simulink model "Struct"  (R2023b)
settings: Solver=VariableStepAuto  StartTime=0.0  StopTime=5  FixedStep=1e-3  MaxStep=1e-3  RelTol=1e-3
values from neighbouring files (symbols this model uses):
  d_1 = 19.4    [CONSTANTS.m]
  d_2 = 24.7    [CONSTANTS.m]
  Ixx_1 = 9.4    [CONSTANTS.m]
  Ixx_2 = 16.5    [CONSTANTS.m]
  Iyy_1 = 9.4    [CONSTANTS.m]
  Iyy_2 = 16.5    [CONSTANTS.m]
  Izz_1 = 0.7    [CONSTANTS.m]
  Izz_2 = 0.7    [CONSTANTS.m]
  Izz_3 = 9.1    [CONSTANTS.m]
  K1_1 = 38.80    (= 38.8)    [CONSTANTS.m]
  K1_2 = 23.30    (= 23.3)    [CONSTANTS.m]
  K2_1 = 2.94    [CONSTANTS.m]
  K2_2 = 2.8    [CONSTANTS.m]
  K3_1 = 9.6    [CONSTANTS.m]
  K3_2 = 11.7    [CONSTANTS.m]
  K4_1 = 0.044    [CONSTANTS.m]
  K4_2 = 0.043    [CONSTANTS.m]
  K5_1 = 15.6    [CONSTANTS.m]
  K5_2 = 9.4    [CONSTANTS.m]
  l_1 = 0.55    [CONSTANTS.m]
  l_2 = 0.55    [CONSTANTS.m]
  m_1 = 46    [CONSTANTS.m]
  m_2 = 78    [CONSTANTS.m]
  x_block = 0.1    [CONSTANTS.m]
  y_block = 0.1    [CONSTANTS.m]
  z_block = 0.1    [CONSTANTS.m]
undefined symbols (not defined in the file or in its folder): X, Y, Z
libraries: sm_lib x19, nesl_utility x13
settings Model: Creator=ycheb  LastModifiedBy=ycheb
settings ExplorerConfigSet: InternalSimMechanicsExplorerSettings="<ExplorerConfiguration><canonicalview>default</canonicalview><AnimationSetting><BasePlaybackSpeed>1.0</BasePlaybackSpeed><PlaybackSpeedFactor>1.0</PlaybackSpeedFactor></AnimationSetting><TilePanel><TileInfo><Tiles Columns=\"1\" Count=\"1\" Rows=\"1\"><Column Weight=\"1\"/><Row Weight=\"1\"/><Tile Height=\"1\" Width=\"1\" X=\"0\" Y=\"0\"/></Tiles></TileInfo><SceneInfo><SceneViewer><BGColor><R>0.60000002384185791</R><G>0.60000002384185791</G><B>0.60000002384185791</B></BGColor><Camera><DoPerspective>off</DoPerspective><Position><X>0.167180391738689205</X><Y>-1.3498377752304076</Y><Z>-0.780521391542822407</Z></Position><Center><X>0.167180391738689205</X><Y>2.22044604925031308e-16</Y><Z>-0.780521391542822407</Z></Center><Up><X>0</X><Y>-0</Y><Z>1</Z></Up><ViewLimDist>1</ViewLimDist><YLim>1.46214565410614039</YLim><XLim>3.24130518896980702</XLim></Camera></SceneViewer></SceneInfo></TilePanel><MechEditorPanel><Cameras/><GfxPanelCameraMap/><VideoCreator><PlaybackSpeedRatio>1.0</PlaybackSpeedRatio><FrameRate>30</FrameRate><VideoFormat>Motion JPEG AVI</VideoFormat><FrameSize>[1280 720]</FrameSize></VideoCreator></MechEditorPanel></ExplorerConfiguration>"

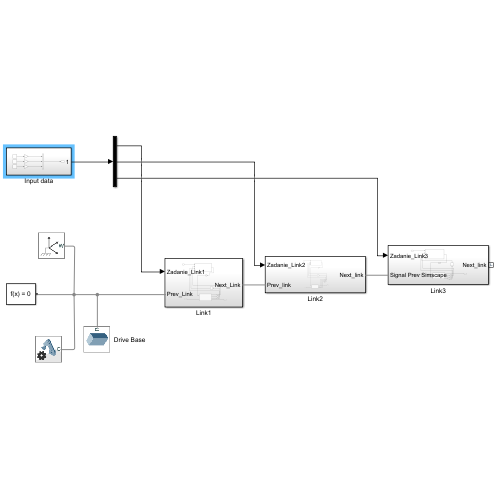
[thumbnail: Simulink's stored preview of the top-level diagram]
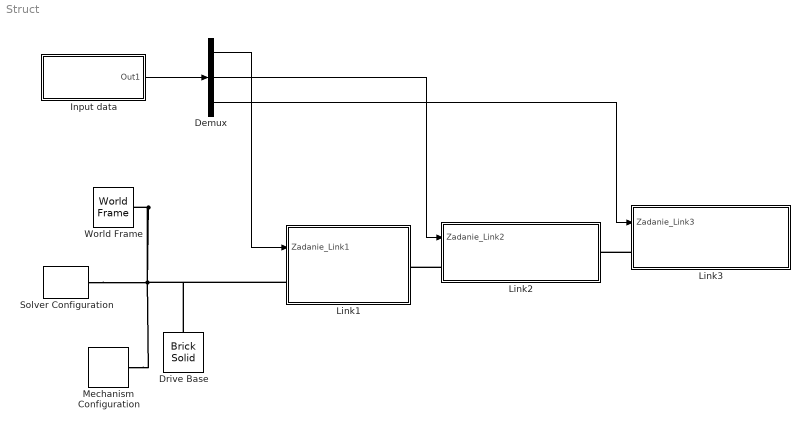
== system Struct ==
  Demux : Demux  Outputs=3
  Drive Base : sm_lib/Body Elements/Brick Solid  GraphicAmbientColor=[0.15 0.15 0.15 1.0]  BasedOnType=Density  BrickDimensions=[x_block y_block z_block]  BrickDimensionsUnits=m  CenterOfMass=[0 0 0]  CenterOfMassUnits=m  GraphicDiffuseColor=[0.5 0.5 0.5]  Density=1000  DensityUnits=kg/m^3  DoExposeReferenceFrame=on  GraphicEmissiveColor=[0.0 0.0 0.0 1.0]  ExportEntireGeometry=off  SerializedFrames=<Frames/>  MarkerShape=Sphere  MarkerSize=10  GraphicType=FromGeometry  InertiaType=CalculateFromGeometry  Mass=1  MassUnits=kg  MomentsOfInertia=[1 1 1]  MomentsOfInertiaUnits=kg*m^2  GraphicOpacity=1.0  ProductsOfInertia=[0 0 0]  ProductsOfInertiaUnits=kg*m^2  GraphicShininess=75  GraphicSpecularColor=[0.5 0.5 0.5 1.0]  GraphicVisPropType=SimpleVisualProperties
  Input data : Subsystem
  Link1 : Subsystem
  Link2 : Subsystem
  Link3 : Subsystem
  Mechanism Configuration : sm_lib/Utilities/Mechanism Configuration  UniformGravity=Constant  GravityVector=[0 0 -9.80665]  GravityVectorUnits=m/s^2  LinearizationDelta=0.001  JointModeTransitionNonlinearIterations=2
  Solver Configuration : nesl_utility/Solver Configuration  PhysicalDomain=network_engine_domain  SubClassName=solver  LeftPortType=input  RightPortType=generic  Tones=[]  Harmonics=[]  SimulateNoise=off  Profile=off  UseLocalSampling=off  EnableSwitchedLinearOptims=on  FrequencyDomain=off  UseCCode=off  RelTol=0.001  AbsTol=0.001  MinStep=1e-09  ToWorkspace=off  RevertToSquareIcSolve=off  NumHomotopyIterations=100  PhasorMode=off  PhasorModeNumHarmonics=1  ConsistencySolver=NEWTON_XTOL_AFTER_FTOL  IndexReductionMethod=DerivativeReplacement  DoDC=off  ResidualTolerance=1e-09  ConsistencyTolSource=GLOBAL  ConsistencyAbsTol=0.001  ConsistencyRelTol=0.001  ConsistencyTolFactor=0.001  UseLocalSolver=off  LocalSolverChoice=NE_BACKWARD_EULER_ADVANCER  ResolveIndetEquations=on  FunctionEvalNumThread=1  LocalSolverSampleTime=0.001  DoFixedCost=off  MaxNonlinIter=3  MaxModeIter=2  ComputeImpulses=off  ImpulseIterations=2  LinearAlgebra=auto  LinearAlgebraNumThread=0  EquationFormulation=NE_TIME_EF  DelaysMemoryBudget=1024  AutomaticFiltering=on  FilteringTimeConstant=0.001  PartitionStorageMethod=AS_NEEDED  PartitionMemoryBudget=1024  PartitionMethod=ROBUST  MultibodyUseLocalSolver=off  MultibodyLocalSolverChoice=ODE1  MultibodyLocalSolverSampleTime=0.001
  World Frame : sm_lib/Frames and Transforms/World Frame
  wires:
  Demux/1 -> Link1/1(Zadanie_Link1)
  Demux/2 -> Link2/1(Zadanie_Link2)
  Demux/3 -> Link3/1(Zadanie_Link3)
  Input data/1(Out1) -> Demux/1
  connections:
  World Frame/RConn1 -- Drive Base/RConn1 -- Link1/LConn1 -- Solver Configuration/RConn1 -- Mechanism Configuration/RConn1
  Link2/LConn1 -- Link1/RConn1
  Link3/LConn1 -- Link2/RConn1

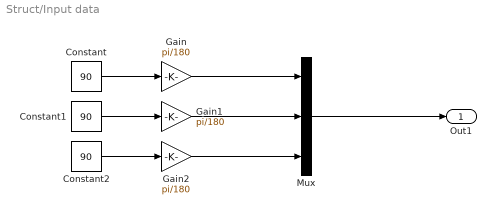
== system Struct/Input data ==
  Constant : Constant  Value=90
  Constant1 : Constant  Value=90
  Constant2 : Constant  Value=90
  Gain : Gain  Gain=pi/180
  Gain1 : Gain  Gain=pi/180
  Gain2 : Gain  Gain=pi/180
  Mux : Mux  Inputs=3
  Out1 : Outport
  wires:
  Mux/1 -> Out1/1
  Constant/1 -> Gain/1
  Constant1/1 -> Gain1/1
  Constant2/1 -> Gain2/1
  Gain/1 -> Mux/1
  Gain1/1 -> Mux/2
  Gain2/1 -> Mux/3

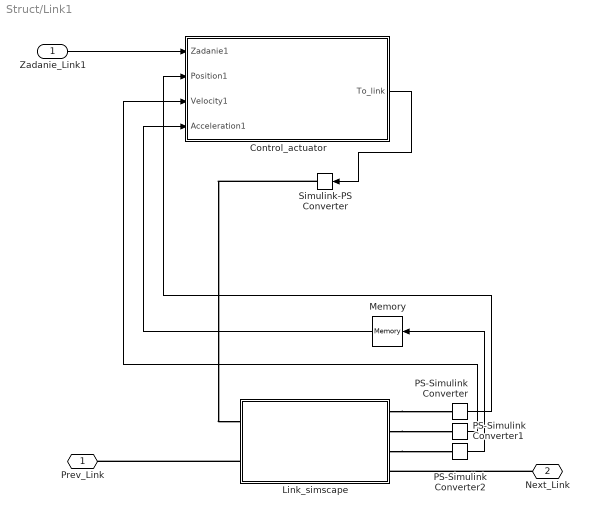
== system Struct/Link1 ==
  Zadanie_Link1 : Inport
  Control_actuator : Subsystem
  Link_simscape : Subsystem
  Memory : Memory
  PS-Simulink Converter : nesl_utility/PS-Simulink Converter  PhysicalDomain=network_engine_domain  SubClassName=ps_output  LeftPortType=input  RightPortType=output  PseudoPeriodic=off  Frequencies=[]  VectorFormat=inherit  Unit=inherit  AffineConversion=off
  PS-Simulink Converter1 : nesl_utility/PS-Simulink Converter  PhysicalDomain=network_engine_domain  SubClassName=ps_output  LeftPortType=input  RightPortType=output  PseudoPeriodic=off  Frequencies=[]  VectorFormat=inherit  Unit=inherit  AffineConversion=off
  PS-Simulink Converter2 : nesl_utility/PS-Simulink Converter  PhysicalDomain=network_engine_domain  SubClassName=ps_output  LeftPortType=input  RightPortType=output  PseudoPeriodic=off  Frequencies=[]  VectorFormat=inherit  Unit=inherit  AffineConversion=off
  Simulink-PS Converter : nesl_utility/Simulink-PS Converter  PhysicalDomain=network_engine_domain  SubClassName=ps_input  LeftPortType=input  RightPortType=output  PseudoPeriodic=off  Frequencies=[]  NoiseDistribution=none  NoiseParameters=[]  Unit=1  AffineConversion=off  FilteringAndDerivatives=provide  SimscapeFilterOrder=1  InputFilterTimeConstant=0.001  UdotUserProvided=0
  Prev_Link : PMIOPort  Side=Left
  Next_Link : PMIOPort  Port=2  Side=Right
  wires:
  Control_actuator/1(To_link) -> Simulink-PS Converter/1
  PS-Simulink Converter/1 -> Control_actuator/2(Position1)
  PS-Simulink Converter1/1 -> Control_actuator/3(Velocity1)
  PS-Simulink Converter2/1 -> Memory/1
  Zadanie_Link1/1 -> Control_actuator/1(Zadanie1)
  Memory/1 -> Control_actuator/4(Acceleration1)
  connections:
  Link_simscape/LConn2 -- Prev_Link/RConn1
  Next_Link/RConn1 -- Link_simscape/RConn4
  Link_simscape/RConn1 -- PS-Simulink Converter/LConn1
  Link_simscape/RConn3 -- PS-Simulink Converter2/LConn1
  Link_simscape/RConn2 -- PS-Simulink Converter1/LConn1
  Simulink-PS Converter/RConn1 -- Link_simscape/LConn1

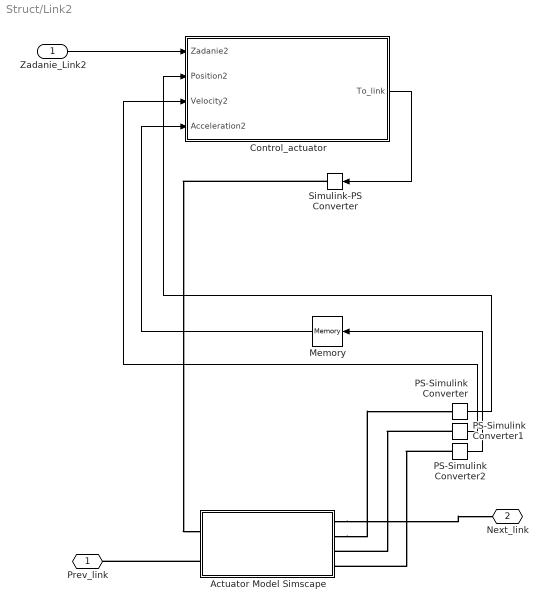
== system Struct/Link2 ==
  Zadanie_Link2 : Inport
  Actuator Model Simscape : Subsystem
  Control_actuator : Subsystem
  Memory : Memory
  PS-Simulink Converter : nesl_utility/PS-Simulink Converter  PhysicalDomain=network_engine_domain  SubClassName=ps_output  LeftPortType=input  RightPortType=output  PseudoPeriodic=off  Frequencies=[]  VectorFormat=inherit  Unit=inherit  AffineConversion=off
  PS-Simulink Converter1 : nesl_utility/PS-Simulink Converter  PhysicalDomain=network_engine_domain  SubClassName=ps_output  LeftPortType=input  RightPortType=output  PseudoPeriodic=off  Frequencies=[]  VectorFormat=inherit  Unit=inherit  AffineConversion=off
  PS-Simulink Converter2 : nesl_utility/PS-Simulink Converter  PhysicalDomain=network_engine_domain  SubClassName=ps_output  LeftPortType=input  RightPortType=output  PseudoPeriodic=off  Frequencies=[]  VectorFormat=inherit  Unit=inherit  AffineConversion=off
  Simulink-PS Converter : nesl_utility/Simulink-PS Converter  PhysicalDomain=network_engine_domain  SubClassName=ps_input  LeftPortType=input  RightPortType=output  PseudoPeriodic=off  Frequencies=[]  NoiseDistribution=none  NoiseParameters=[]  Unit=1  AffineConversion=off  FilteringAndDerivatives=provide  SimscapeFilterOrder=1  InputFilterTimeConstant=0.001  UdotUserProvided=0
  Prev_link : PMIOPort  Side=Left
  Next_link : PMIOPort  Port=2  Side=Right
  wires:
  PS-Simulink Converter2/1 -> Memory/1
  PS-Simulink Converter/1 -> Control_actuator/2(Position2)
  PS-Simulink Converter1/1 -> Control_actuator/3(Velocity2)
  Control_actuator/1(To_link) -> Simulink-PS Converter/1
  Zadanie_Link2/1 -> Control_actuator/1(Zadanie2)
  Memory/1 -> Control_actuator/4(Acceleration2)
  connections:
  Actuator Model Simscape/LConn2 -- Prev_link/RConn1
  PS-Simulink Converter1/LConn1 -- Actuator Model Simscape/RConn3
  PS-Simulink Converter2/LConn1 -- Actuator Model Simscape/RConn4
  Actuator Model Simscape/RConn1 -- Next_link/RConn1
  Actuator Model Simscape/RConn2 -- PS-Simulink Converter/LConn1
  Simulink-PS Converter/RConn1 -- Actuator Model Simscape/LConn1

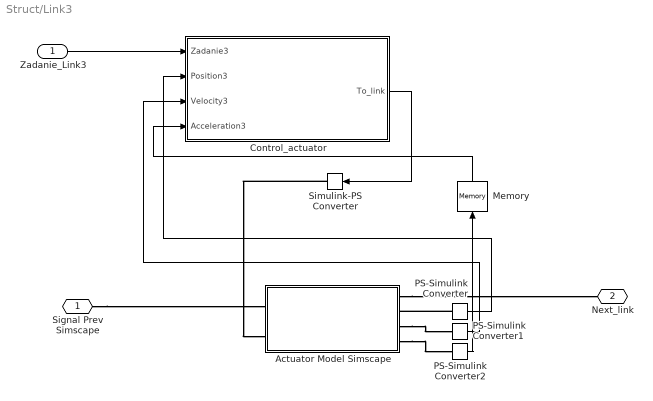
== system Struct/Link3 ==
  Zadanie_Link3 : Inport
  Actuator Model Simscape : Subsystem
  Control_actuator : Subsystem
  Memory : Memory
  PS-Simulink Converter : nesl_utility/PS-Simulink Converter  PhysicalDomain=network_engine_domain  SubClassName=ps_output  LeftPortType=input  RightPortType=output  PseudoPeriodic=off  Frequencies=[]  VectorFormat=inherit  Unit=inherit  AffineConversion=off
  PS-Simulink Converter1 : nesl_utility/PS-Simulink Converter  PhysicalDomain=network_engine_domain  SubClassName=ps_output  LeftPortType=input  RightPortType=output  PseudoPeriodic=off  Frequencies=[]  VectorFormat=inherit  Unit=inherit  AffineConversion=off
  PS-Simulink Converter2 : nesl_utility/PS-Simulink Converter  PhysicalDomain=network_engine_domain  SubClassName=ps_output  LeftPortType=input  RightPortType=output  PseudoPeriodic=off  Frequencies=[]  VectorFormat=inherit  Unit=inherit  AffineConversion=off
  Simulink-PS Converter : nesl_utility/Simulink-PS Converter  PhysicalDomain=network_engine_domain  SubClassName=ps_input  LeftPortType=input  RightPortType=output  PseudoPeriodic=off  Frequencies=[]  NoiseDistribution=none  NoiseParameters=[]  Unit=1  AffineConversion=off  FilteringAndDerivatives=provide  SimscapeFilterOrder=1  InputFilterTimeConstant=0.001  UdotUserProvided=0
  Signal Prev Simscape : PMIOPort  Side=Left
  Next_link : PMIOPort  Port=2  Side=Right
  wires:
  Zadanie_Link3/1 -> Control_actuator/1(Zadanie3)
  Control_actuator/1(To_link) -> Simulink-PS Converter/1
  PS-Simulink Converter/1 -> Control_actuator/2(Position3)
  PS-Simulink Converter1/1 -> Control_actuator/3(Velocity3)
  PS-Simulink Converter2/1 -> Memory/1
  Memory/1 -> Control_actuator/4(Acceleration3)
  connections:
  Signal Prev Simscape/RConn1 -- Actuator Model Simscape/LConn1
  PS-Simulink Converter/LConn1 -- Actuator Model Simscape/RConn2
  Actuator Model Simscape/RConn3 -- PS-Simulink Converter1/LConn1
  Actuator Model Simscape/RConn4 -- PS-Simulink Converter2/LConn1
  Actuator Model Simscape/RConn1 -- Next_link/RConn1
  Simulink-PS Converter/RConn1 -- Actuator Model Simscape/LConn2

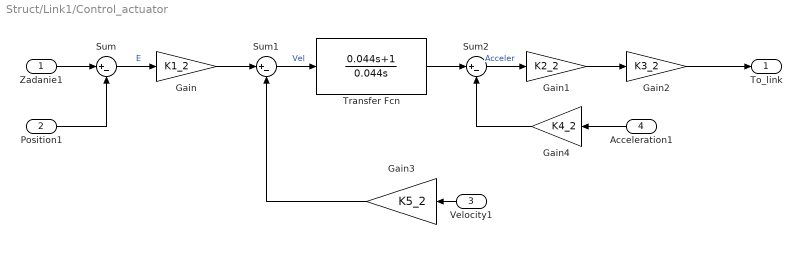
== system Struct/Link1/Control_actuator ==
  Zadanie1 : Inport
  Position1 : Inport  Port=2
  Velocity1 : Inport  Port=3
  Acceleration1 : Inport  Port=4
  Gain : Gain  Gain=K1_2
  Gain1 : Gain  Gain=K2_2
  Gain2 : Gain  Gain=K3_2
  Gain3 : Gain  Gain=K5_2
  Gain4 : Gain  Gain=K4_2
  Sum : Sum  Inputs=|+-
  Sum1 : Sum  Inputs=|+-
  Sum2 : Sum  Inputs=|+-
  Transfer Fcn : TransferFcn  Numerator=[0.044 1]  Denominator=[0.044 0]
  To_link : Outport
  wires:
  Velocity1/1 -> Gain3/1
  Sum/1 -> Gain/1  "E"
  Gain/1 -> Sum1/1
  Transfer Fcn/1 -> Sum2/1
  Gain4/1 -> Sum2/2
  Sum1/1 -> Transfer Fcn/1  "Vel"
  Gain1/1 -> Gain2/1
  Sum2/1 -> Gain1/1  "Acceler"
  Zadanie1/1 -> Sum/1
  Acceleration1/1 -> Gain4/1
  Gain2/1 -> To_link/1
  Position1/1 -> Sum/2
  Gain3/1 -> Sum1/2

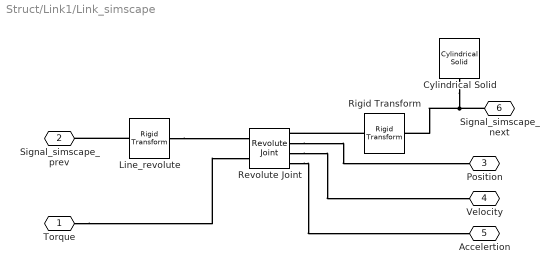
== system Struct/Link1/Link_simscape ==
  Cylindrical Solid : sm_lib/Body Elements/Cylindrical Solid  GraphicAmbientColor=[0.15 0.15 0.15 1.0]  BasedOnType=Density  CenterOfMass=[0 0 0]  CenterOfMassUnits=m  GraphicDiffuseColor=[0.5 0.5 0.5]  CylinderLength=l_2  CylinderLengthUnits=m  CylinderRadius=d_2/2  CylinderRadiusUnits=cm  Density=1000  DensityUnits=kg/m^3  DoExposeReferenceFrame=on  GraphicEmissiveColor=[0.0 0.0 0.0 1.0]  ExportEntireGeometry=off  SerializedFrames=<Frames/>  MarkerShape=Sphere  MarkerSize=10  GraphicType=FromGeometry  InertiaType=Custom  Mass=m_2  MassUnits=kg  MomentsOfInertia=[Ixx_2 Iyy_2 Izz_2]  MomentsOfInertiaUnits=kg*m^2  GraphicOpacity=1.0  ProductsOfInertia=[0 0 0]  ProductsOfInertiaUnits=kg*m^2  GraphicShininess=75  GraphicSpecularColor=[0.5 0.5 0.5 1.0]  GraphicVisPropType=SimpleVisualProperties
  Line_revolute : sm_lib/Frames and Transforms/Rigid Transform  TranslationMethod=Cartesian  TranslationStandardOffset=0  TranslationStandardOffsetUnits=m  TranslationStandardAxis=+Z  TranslationCartesianOffset=[0 0 -z_block/2]  TranslationCartesianOffsetUnits=m  TranslationROffset=0  TranslationROffsetUnits=m  TranslationZOffset=0  TranslationZOffsetUnits=m  TranslationThetaOffset=0  TranslationThetaOffsetUnits=deg  RotationMethod=StandardAxis  RotationAngleUnits=deg  RotationStandardAxis=+X  RotationAngle=90  RotationArbitraryAxis=[0 0 1]  FollAlignAxisA=+X  BaseAlignAxisA=+Y  FollAlignAxisB=+Y  BaseAlignAxisB=+Z  RotationSequenceAxes=FollowerAxes  RotationSequence=XYX  RotationSequenceAngles=[0 0 0]  RotationSequenceAnglesUnits=deg  RotationMatrix=[1 0 0; 0 1 0; 0 0 1]  Quaternion=[1 0 0 0]
  Revolute Joint : sm_lib/Joints/Revolute Joint  JointMode=Normal  SenseConstraintForce=off  SenseConstraintForceX=off  SenseConstraintForceY=off  SenseConstraintForceZ=off  SenseConstraintTorque=off  SenseConstraintTorqueX=off  SenseConstraintTorqueY=off  SenseConstraintTorqueZ=off  SenseTotalForce=off  SenseTotalForceX=off  SenseTotalForceY=off  SenseTotalForceZ=off  SenseTotalTorque=off  SenseTotalTorqueX=off  SenseTotalTorqueY=off  SenseTotalTorqueZ=off  CompositeWrenchDir=FollowerOnBase  CompositeWrenchFrame=BaseFrame  EquilibriumPosition=0  EquilibriumPositionUnits=deg  SpringStiffness=0  SpringStiffnessUnits=N*m/deg  DampingCoefficient=0  DampingCoefficientUnits=N*m/(deg/s)  TorqueActuationMode=InputTorque  MotionActuationMode=ComputedMotion  SensePosition=on  SenseVelocity=on  SenseAcceleration=on  SenseTorqueForce=off  SenseLowerLimitTorqueForce=off  SenseUpperLimitTorqueForce=off  LowerLimitSpecify=on  LowerLimitBound=-50  LowerLimitBoundUnits=deg  LowerLimitStiffness=2000000  LowerLimitStiffnessUnits=N*m/deg  LowerLimitDamping=100000  LowerLimitDampingUnits=N*m/(deg/s)  LowerLimitTransitionRegionWidth=0.1  LowerLimitTransitionRegionWidthUnits=deg  UpperLimitSpecify=on  UpperLimitBound=50  UpperLimitBoundUnits=deg  UpperLimitStiffness=2000000  UpperLimitStiffnessUnits=N*m/deg  UpperLimitDamping=100000  UpperLimitDampingUnits=N*m/(deg/s)  UpperLimitTransitionRegionWidth=0.1  UpperLimitTransitionRegionWidthUnits=deg  PositionTargetSpecify=off  PositionTargetPriority=High  PositionTargetValue=15  PositionTargetValueUnits=deg  VelocityTargetSpecify=off  VelocityTargetPriority=High  VelocityTargetValue=0  VelocityTargetValueUnits=deg/s
  Rigid Transform : sm_lib/Frames and Transforms/Rigid Transform  TranslationMethod=Cartesian  TranslationStandardOffset=0  TranslationStandardOffsetUnits=m  TranslationStandardAxis=+Z  TranslationCartesianOffset=[0 -l_2 / 2 0]  TranslationCartesianOffsetUnits=m  TranslationROffset=0  TranslationROffsetUnits=m  TranslationZOffset=0  TranslationZOffsetUnits=m  TranslationThetaOffset=0  TranslationThetaOffsetUnits=deg  RotationMethod=StandardAxis  RotationAngleUnits=deg  RotationStandardAxis=+X  RotationAngle=90  RotationArbitraryAxis=[0 0 1]  FollAlignAxisA=+X  BaseAlignAxisA=+Y  FollAlignAxisB=+Y  BaseAlignAxisB=+Z  RotationSequenceAxes=FollowerAxes  RotationSequence=XYX  RotationSequenceAngles=[0 0 0]  RotationSequenceAnglesUnits=deg  RotationMatrix=[1 0 0; 0 1 0; 0 0 1]  Quaternion=[1 0 0 0]
  Torque : PMIOPort  Side=Left
  Signal_simscape_prev : PMIOPort  Port=2  Side=Left
  Position : PMIOPort  Port=3  Side=Right
  Velocity : PMIOPort  Port=4  Side=Right
  Accelertion : PMIOPort  Port=5  Side=Right
  Signal_simscape_next : PMIOPort  Port=6  Side=Right
  connections:
  Rigid Transform/LConn1 -- Revolute Joint/RConn1
  Signal_simscape_next/RConn1 -- Rigid Transform/RConn1 -- Cylindrical Solid/RConn1
  Line_revolute/LConn1 -- Signal_simscape_prev/RConn1
  Line_revolute/RConn1 -- Revolute Joint/LConn1
  Torque/RConn1 -- Revolute Joint/LConn2
  Revolute Joint/RConn2 -- Position/RConn1
  Revolute Joint/RConn3 -- Velocity/RConn1
  Revolute Joint/RConn4 -- Accelertion/RConn1

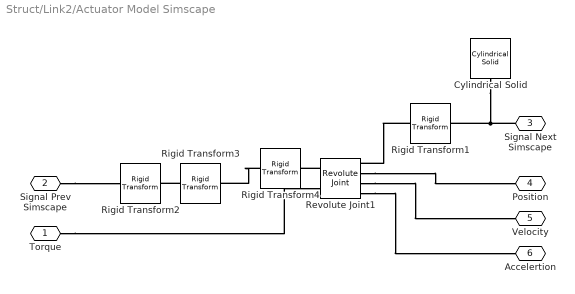
== system Struct/Link2/Actuator Model Simscape ==
  Cylindrical Solid : sm_lib/Body Elements/Cylindrical Solid  GraphicAmbientColor=[0.15 0.15 0.15 1.0]  BasedOnType=Density  CenterOfMass=[0 0 0]  CenterOfMassUnits=m  GraphicDiffuseColor=[0.5 0.5 0.5]  CylinderLength=l_1  CylinderLengthUnits=m  CylinderRadius=d_1 / 2  CylinderRadiusUnits=cm  Density=1000  DensityUnits=kg/m^3  DoExposeReferenceFrame=on  GraphicEmissiveColor=[0.0 0.0 0.0 1.0]  ExportEntireGeometry=off  SerializedFrames=<Frames/>  MarkerShape=Sphere  MarkerSize=10  GraphicType=FromGeometry  InertiaType=Custom  Mass=m_1  MassUnits=kg  MomentsOfInertia=[Ixx_1 Iyy_1 Izz_1]  MomentsOfInertiaUnits=kg*m^2  GraphicOpacity=1.0  ProductsOfInertia=[0 0 0]  ProductsOfInertiaUnits=kg*m^2  GraphicShininess=75  GraphicSpecularColor=[0.5 0.5 0.5 1.0]  GraphicVisPropType=SimpleVisualProperties
  Revolute Joint1 : sm_lib/Joints/Revolute Joint  JointMode=Normal  SenseConstraintForce=off  SenseConstraintForceX=off  SenseConstraintForceY=off  SenseConstraintForceZ=off  SenseConstraintTorque=off  SenseConstraintTorqueX=off  SenseConstraintTorqueY=off  SenseConstraintTorqueZ=off  SenseTotalForce=off  SenseTotalForceX=off  SenseTotalForceY=off  SenseTotalForceZ=off  SenseTotalTorque=off  SenseTotalTorqueX=off  SenseTotalTorqueY=off  SenseTotalTorqueZ=off  CompositeWrenchDir=FollowerOnBase  CompositeWrenchFrame=BaseFrame  EquilibriumPosition=0  EquilibriumPositionUnits=deg  SpringStiffness=0  SpringStiffnessUnits=N*m/deg  DampingCoefficient=0  DampingCoefficientUnits=N*m/(deg/s)  TorqueActuationMode=InputTorque  MotionActuationMode=ComputedMotion  SensePosition=on  SenseVelocity=on  SenseAcceleration=on  SenseTorqueForce=off  SenseLowerLimitTorqueForce=off  SenseUpperLimitTorqueForce=off  LowerLimitSpecify=on  LowerLimitBound=-30  LowerLimitBoundUnits=deg  LowerLimitStiffness=2000000  LowerLimitStiffnessUnits=N*m/deg  LowerLimitDamping=100000  LowerLimitDampingUnits=N*m/(deg/s)  LowerLimitTransitionRegionWidth=0.1  LowerLimitTransitionRegionWidthUnits=deg  UpperLimitSpecify=on  UpperLimitBound=30  UpperLimitBoundUnits=deg  UpperLimitStiffness=2000000  UpperLimitStiffnessUnits=N*m/deg  UpperLimitDamping=100000  UpperLimitDampingUnits=N*m/(deg/s)  UpperLimitTransitionRegionWidth=0.1  UpperLimitTransitionRegionWidthUnits=deg  PositionTargetSpecify=off  PositionTargetPriority=High  PositionTargetValue=0  PositionTargetValueUnits=deg  VelocityTargetSpecify=off  VelocityTargetPriority=High  VelocityTargetValue=0  VelocityTargetValueUnits=deg/s
  Rigid Transform1 : sm_lib/Frames and Transforms/Rigid Transform  TranslationMethod=Cartesian  TranslationStandardOffset=0  TranslationStandardOffsetUnits=m  TranslationStandardAxis=+Z  TranslationCartesianOffset=[0 l_1 / 2 0]  TranslationCartesianOffsetUnits=m  TranslationROffset=0  TranslationROffsetUnits=m  TranslationZOffset=0  TranslationZOffsetUnits=m  TranslationThetaOffset=0  TranslationThetaOffsetUnits=deg  RotationMethod=StandardAxis  RotationAngleUnits=deg  RotationStandardAxis=+X  RotationAngle=90  RotationArbitraryAxis=[0 0 1]  FollAlignAxisA=+X  BaseAlignAxisA=+Y  FollAlignAxisB=+Y  BaseAlignAxisB=+Z  RotationSequenceAxes=FollowerAxes  RotationSequence=XYX  RotationSequenceAngles=[0 0 0]  RotationSequenceAnglesUnits=deg  RotationMatrix=[1 0 0; 0 1 0; 0 0 1]  Quaternion=[1 0 0 0]
  Rigid Transform2 : sm_lib/Frames and Transforms/Rigid Transform  TranslationMethod=Cartesian  TranslationStandardOffset=0  TranslationStandardOffsetUnits=m  TranslationStandardAxis=+Z  TranslationCartesianOffset=[0 0 l_1/2]  TranslationCartesianOffsetUnits=m  TranslationROffset=0  TranslationROffsetUnits=m  TranslationZOffset=0  TranslationZOffsetUnits=m  TranslationThetaOffset=0  TranslationThetaOffsetUnits=deg  RotationMethod=None  RotationAngleUnits=deg  RotationStandardAxis=+Y  RotationAngle=90  RotationArbitraryAxis=[0 0 1]  FollAlignAxisA=+X  BaseAlignAxisA=+Y  FollAlignAxisB=+Y  BaseAlignAxisB=+Z  RotationSequenceAxes=FollowerAxes  RotationSequence=XYX  RotationSequenceAngles=[0 0 0]  RotationSequenceAnglesUnits=deg  RotationMatrix=[1 0 0; 0 1 0; 0 0 1]  Quaternion=[1 0 0 0]
  Rigid Transform3 : sm_lib/Frames and Transforms/Rigid Transform  TranslationMethod=None  TranslationStandardOffset=0  TranslationStandardOffsetUnits=m  TranslationStandardAxis=+Z  TranslationCartesianOffset=[0 0 0]  TranslationCartesianOffsetUnits=m  TranslationROffset=0  TranslationROffsetUnits=m  TranslationZOffset=0  TranslationZOffsetUnits=m  TranslationThetaOffset=0  TranslationThetaOffsetUnits=deg  RotationMethod=StandardAxis  RotationAngleUnits=deg  RotationStandardAxis=+X  RotationAngle=90  RotationArbitraryAxis=[0 0 1]  FollAlignAxisA=+X  BaseAlignAxisA=+Y  FollAlignAxisB=+Y  BaseAlignAxisB=+Z  RotationSequenceAxes=FollowerAxes  RotationSequence=XYX  RotationSequenceAngles=[0 0 0]  RotationSequenceAnglesUnits=deg  RotationMatrix=[1 0 0; 0 1 0; 0 0 1]  Quaternion=[1 0 0 0]
  Rigid Transform4 : sm_lib/Frames and Transforms/Rigid Transform  TranslationMethod=None  TranslationStandardOffset=0  TranslationStandardOffsetUnits=m  TranslationStandardAxis=+Z  TranslationCartesianOffset=[0 0 0]  TranslationCartesianOffsetUnits=m  TranslationROffset=0  TranslationROffsetUnits=m  TranslationZOffset=0  TranslationZOffsetUnits=m  TranslationThetaOffset=0  TranslationThetaOffsetUnits=deg  RotationMethod=StandardAxis  RotationAngleUnits=deg  RotationStandardAxis=+Y  RotationAngle=180  RotationArbitraryAxis=[0 0 1]  FollAlignAxisA=+X  BaseAlignAxisA=+Y  FollAlignAxisB=+Y  BaseAlignAxisB=+Z  RotationSequenceAxes=FollowerAxes  RotationSequence=XYX  RotationSequenceAngles=[0 0 0]  RotationSequenceAnglesUnits=deg  RotationMatrix=[1 0 0; 0 1 0; 0 0 1]  Quaternion=[1 0 0 0]
  Torque : PMIOPort  Side=Left
  Signal Prev Simscape : PMIOPort  Port=2  Side=Left
  Signal Next Simscape : PMIOPort  Port=3  Side=Right
  Position : PMIOPort  Port=4  Side=Right
  Velocity : PMIOPort  Port=5  Side=Right
  Accelertion : PMIOPort  Port=6  Side=Right
  connections:
  Revolute Joint1/LConn1 -- Rigid Transform4/RConn1
  Signal Next Simscape/RConn1 -- Cylindrical Solid/RConn1 -- Rigid Transform1/RConn1
  Signal Prev Simscape/RConn1 -- Rigid Transform2/LConn1
  Rigid Transform1/LConn1 -- Revolute Joint1/RConn1
  Rigid Transform3/LConn1 -- Rigid Transform2/RConn1
  Revolute Joint1/RConn2 -- Position/RConn1
  Revolute Joint1/RConn3 -- Velocity/RConn1
  Revolute Joint1/RConn4 -- Accelertion/RConn1
  Torque/RConn1 -- Revolute Joint1/LConn2
  Rigid Transform4/LConn1 -- Rigid Transform3/RConn1

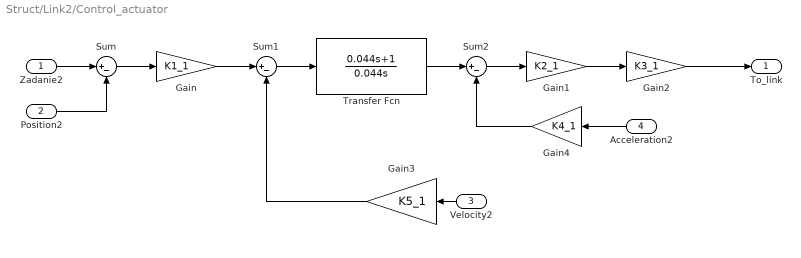
== system Struct/Link2/Control_actuator ==
  Zadanie2 : Inport
  Position2 : Inport  Port=2
  Velocity2 : Inport  Port=3
  Acceleration2 : Inport  Port=4
  Gain : Gain  Gain=K1_1
  Gain1 : Gain  Gain=K2_1
  Gain2 : Gain  Gain=K3_1
  Gain3 : Gain  Gain=K5_1
  Gain4 : Gain  Gain=K4_1
  Sum : Sum  Inputs=|+-
  Sum1 : Sum  Inputs=|+-
  Sum2 : Sum  Inputs=|+-
  Transfer Fcn : TransferFcn  Numerator=[0.044 1]  Denominator=[0.044 0]
  To_link : Outport
  wires:
  Velocity2/1 -> Gain3/1
  Sum/1 -> Gain/1
  Gain/1 -> Sum1/1
  Transfer Fcn/1 -> Sum2/1
  Gain4/1 -> Sum2/2
  Sum1/1 -> Transfer Fcn/1
  Gain3/1 -> Sum1/2
  Gain1/1 -> Gain2/1
  Position2/1 -> Sum/2
  Sum2/1 -> Gain1/1
  Zadanie2/1 -> Sum/1
  Acceleration2/1 -> Gain4/1
  Gain2/1 -> To_link/1

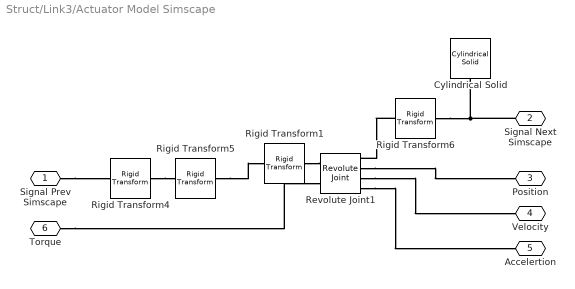
== system Struct/Link3/Actuator Model Simscape ==
  Cylindrical Solid : sm_lib/Body Elements/Cylindrical Solid  GraphicAmbientColor=[0.15 0.15 0.15 1.0]  BasedOnType=Density  CenterOfMass=[0 0 0]  CenterOfMassUnits=m  GraphicDiffuseColor=[0.5 0.5 0.5]  CylinderLength=l_2  CylinderLengthUnits=m  CylinderRadius=d_2 / 2  CylinderRadiusUnits=cm  Density=1000  DensityUnits=kg/m^3  DoExposeReferenceFrame=on  GraphicEmissiveColor=[0.0 0.0 0.0 1.0]  ExportEntireGeometry=off  SerializedFrames=<Frames/>  MarkerShape=Sphere  MarkerSize=10  GraphicType=FromGeometry  InertiaType=Custom  Mass=m_2  MassUnits=kg  MomentsOfInertia=[Ixx_2 Iyy_2 Izz_3]  MomentsOfInertiaUnits=kg*m^2  GraphicOpacity=1.0  ProductsOfInertia=[0 0 0]  ProductsOfInertiaUnits=kg*m^2  GraphicShininess=75  GraphicSpecularColor=[0.5 0.5 0.5 1.0]  GraphicVisPropType=SimpleVisualProperties
  Revolute Joint1 : sm_lib/Joints/Revolute Joint  JointMode=Normal  SenseConstraintForce=off  SenseConstraintForceX=off  SenseConstraintForceY=off  SenseConstraintForceZ=off  SenseConstraintTorque=off  SenseConstraintTorqueX=off  SenseConstraintTorqueY=off  SenseConstraintTorqueZ=off  SenseTotalForce=off  SenseTotalForceX=off  SenseTotalForceY=off  SenseTotalForceZ=off  SenseTotalTorque=off  SenseTotalTorqueX=off  SenseTotalTorqueY=off  SenseTotalTorqueZ=off  CompositeWrenchDir=FollowerOnBase  CompositeWrenchFrame=BaseFrame  EquilibriumPosition=0  EquilibriumPositionUnits=deg  SpringStiffness=0  SpringStiffnessUnits=N*m/deg  DampingCoefficient=0  DampingCoefficientUnits=N*m/(deg/s)  TorqueActuationMode=InputTorque  MotionActuationMode=ComputedMotion  SensePosition=on  SenseVelocity=on  SenseAcceleration=on  SenseTorqueForce=off  SenseLowerLimitTorqueForce=off  SenseUpperLimitTorqueForce=off  LowerLimitSpecify=on  LowerLimitBound=-15  LowerLimitBoundUnits=deg  LowerLimitStiffness=2000000  LowerLimitStiffnessUnits=N*m/deg  LowerLimitDamping=100000  LowerLimitDampingUnits=N*m/(deg/s)  LowerLimitTransitionRegionWidth=0.1  LowerLimitTransitionRegionWidthUnits=deg  UpperLimitSpecify=on  UpperLimitBound=15  UpperLimitBoundUnits=deg  UpperLimitStiffness=2000000  UpperLimitStiffnessUnits=N*m/deg  UpperLimitDamping=100000  UpperLimitDampingUnits=N*m/(deg/s)  UpperLimitTransitionRegionWidth=0.1  UpperLimitTransitionRegionWidthUnits=deg  PositionTargetSpecify=off  PositionTargetPriority=High  PositionTargetValue=30  PositionTargetValueUnits=deg  VelocityTargetSpecify=off  VelocityTargetPriority=High  VelocityTargetValue=0  VelocityTargetValueUnits=deg/s
  Rigid Transform1 : sm_lib/Frames and Transforms/Rigid Transform  TranslationMethod=None  TranslationStandardOffset=0  TranslationStandardOffsetUnits=m  TranslationStandardAxis=+Z  TranslationCartesianOffset=[0 0 0]  TranslationCartesianOffsetUnits=m  TranslationROffset=0  TranslationROffsetUnits=m  TranslationZOffset=0  TranslationZOffsetUnits=m  TranslationThetaOffset=0  TranslationThetaOffsetUnits=deg  RotationMethod=StandardAxis  RotationAngleUnits=deg  RotationStandardAxis=+Y  RotationAngle=180  RotationArbitraryAxis=[0 0 1]  FollAlignAxisA=+X  BaseAlignAxisA=+Y  FollAlignAxisB=+Y  BaseAlignAxisB=+Z  RotationSequenceAxes=FollowerAxes  RotationSequence=XYX  RotationSequenceAngles=[0 0 0]  RotationSequenceAnglesUnits=deg  RotationMatrix=[1 0 0; 0 1 0; 0 0 1]  Quaternion=[1 0 0 0]
  Rigid Transform4 : sm_lib/Frames and Transforms/Rigid Transform  TranslationMethod=Cartesian  TranslationStandardOffset=0  TranslationStandardOffsetUnits=m  TranslationStandardAxis=+Z  TranslationCartesianOffset=[0 0 -l_1 / 2]  TranslationCartesianOffsetUnits=m  TranslationROffset=0  TranslationROffsetUnits=m  TranslationZOffset=0  TranslationZOffsetUnits=m  TranslationThetaOffset=0  TranslationThetaOffsetUnits=deg  RotationMethod=None  RotationAngleUnits=deg  RotationStandardAxis=+Z  RotationAngle=0.0  RotationArbitraryAxis=[0 0 1]  FollAlignAxisA=+X  BaseAlignAxisA=+Y  FollAlignAxisB=+Y  BaseAlignAxisB=+Z  RotationSequenceAxes=FollowerAxes  RotationSequence=XYX  RotationSequenceAngles=[0 0 0]  RotationSequenceAnglesUnits=deg  RotationMatrix=[1 0 0; 0 1 0; 0 0 1]  Quaternion=[1 0 0 0]
  Rigid Transform5 : sm_lib/Frames and Transforms/Rigid Transform  TranslationMethod=None  TranslationStandardOffset=0  TranslationStandardOffsetUnits=m  TranslationStandardAxis=+Z  TranslationCartesianOffset=[0 0 0]  TranslationCartesianOffsetUnits=m  TranslationROffset=0  TranslationROffsetUnits=m  TranslationZOffset=0  TranslationZOffsetUnits=m  TranslationThetaOffset=0  TranslationThetaOffsetUnits=deg  RotationMethod=StandardAxis  RotationAngleUnits=deg  RotationStandardAxis=+X  RotationAngle=90  RotationArbitraryAxis=[0 0 1]  FollAlignAxisA=+X  BaseAlignAxisA=+Y  FollAlignAxisB=+Y  BaseAlignAxisB=+Z  RotationSequenceAxes=FollowerAxes  RotationSequence=XYX  RotationSequenceAngles=[0 0 0]  RotationSequenceAnglesUnits=deg  RotationMatrix=[1 0 0; 0 1 0; 0 0 1]  Quaternion=[1 0 0 0]
  Rigid Transform6 : sm_lib/Frames and Transforms/Rigid Transform  TranslationMethod=Cartesian  TranslationStandardOffset=0  TranslationStandardOffsetUnits=m  TranslationStandardAxis=+Z  TranslationCartesianOffset=[0 -l_2 / 2 0]  TranslationCartesianOffsetUnits=m  TranslationROffset=0  TranslationROffsetUnits=m  TranslationZOffset=0  TranslationZOffsetUnits=m  TranslationThetaOffset=0  TranslationThetaOffsetUnits=deg  RotationMethod=StandardAxis  RotationAngleUnits=deg  RotationStandardAxis=+X  RotationAngle=90  RotationArbitraryAxis=[0 0 1]  FollAlignAxisA=+X  BaseAlignAxisA=+Y  FollAlignAxisB=+Y  BaseAlignAxisB=+Z  RotationSequenceAxes=FollowerAxes  RotationSequence=XYX  RotationSequenceAngles=[0 0 0]  RotationSequenceAnglesUnits=deg  RotationMatrix=[1 0 0; 0 1 0; 0 0 1]  Quaternion=[1 0 0 0]
  Signal Prev Simscape : PMIOPort  Side=Left
  Signal Next Simscape : PMIOPort  Port=2  Side=Right
  Position : PMIOPort  Port=3  Side=Right
  Velocity : PMIOPort  Port=4  Side=Right
  Accelertion : PMIOPort  Port=5  Side=Right
  Torque : PMIOPort  Port=6  Side=Left
  connections:
  Rigid Transform5/RConn1 -- Rigid Transform1/LConn1
  Rigid Transform6/LConn1 -- Revolute Joint1/RConn1
  Revolute Joint1/RConn2 -- Position/RConn1
  Revolute Joint1/RConn3 -- Velocity/RConn1
  Revolute Joint1/RConn4 -- Accelertion/RConn1
  Torque/RConn1 -- Revolute Joint1/LConn2
  Rigid Transform4/RConn1 -- Rigid Transform5/LConn1
  Signal Prev Simscape/RConn1 -- Rigid Transform4/LConn1
  Rigid Transform6/RConn1 -- Signal Next Simscape/RConn1 -- Cylindrical Solid/RConn1
  Rigid Transform1/RConn1 -- Revolute Joint1/LConn1

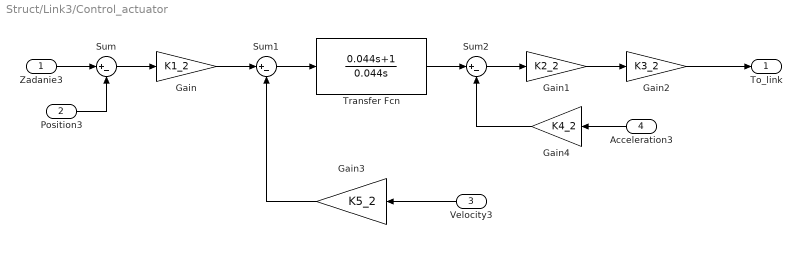
== system Struct/Link3/Control_actuator ==
  Zadanie3 : Inport
  Position3 : Inport  Port=2
  Velocity3 : Inport  Port=3
  Acceleration3 : Inport  Port=4
  Gain : Gain  Gain=K1_2
  Gain1 : Gain  Gain=K2_2
  Gain2 : Gain  Gain=K3_2
  Gain3 : Gain  Gain=K5_2
  Gain4 : Gain  Gain=K4_2
  Sum : Sum  Inputs=|+-
  Sum1 : Sum  Inputs=|+-
  Sum2 : Sum  Inputs=|+-
  Transfer Fcn : TransferFcn  Numerator=[0.044 1]  Denominator=[0.044 0]
  To_link : Outport
  wires:
  Velocity3/1 -> Gain3/1
  Sum/1 -> Gain/1
  Gain/1 -> Sum1/1
  Transfer Fcn/1 -> Sum2/1
  Gain4/1 -> Sum2/2
  Sum1/1 -> Transfer Fcn/1
  Gain3/1 -> Sum1/2
  Gain1/1 -> Gain2/1
  Position3/1 -> Sum/2
  Sum2/1 -> Gain1/1
  Zadanie3/1 -> Sum/1
  Acceleration3/1 -> Gain4/1
  Gain2/1 -> To_link/1
